simulink model "DatAnalysis"  (R2020a)
settings: Solver=FixedStepAuto  StartTime=0.0  StopTime=t_end  FixedStep=0.001  RelTol=1e-3
undefined symbols (not defined in the file or in its folder): DiscIntNeverNeededParam, Je, Ka, Ks, Le, We
libraries: simulink x6, dspstat3 x2, simulink_extras x2, dspsigops x2
settings Model: Creator=leona  LastModifiedBy=leona
settings DataIOCC: SaveFormat=StructureWithTime  SaveOutput=off  SignalLogging=off  DSMLogging=off  SaveTime=off  ReturnWorkspaceOutputs=off

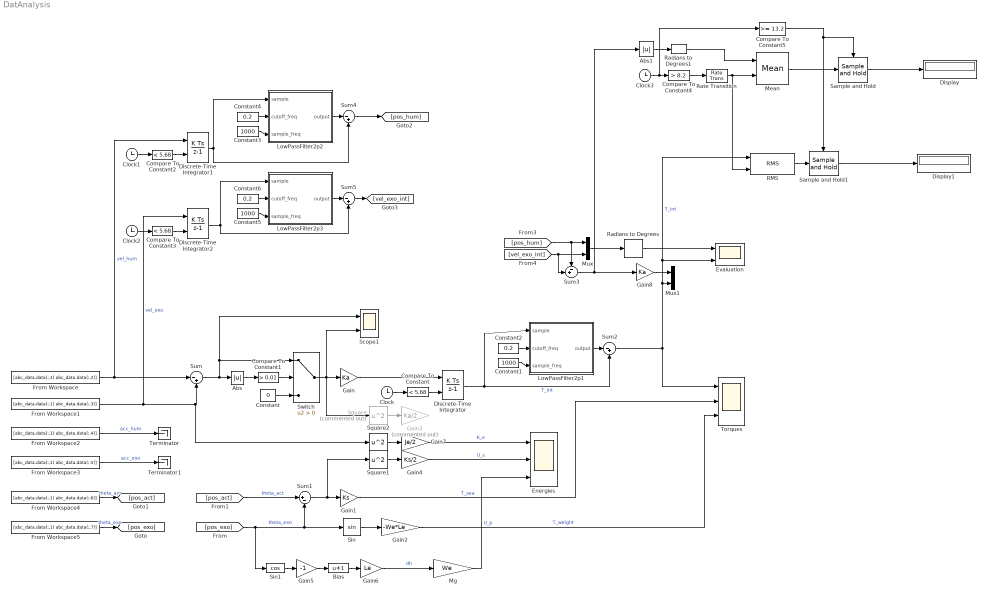
== system DatAnalysis ==
  Abs : Abs
  Abs1 : Abs
  Bias : Bias  Bias=1
  Clock{,1..3} (4 alike) : Clock
  Compare To Constant : simulink/Logic and Bit Operations/Compare To Constant  relop=<  const=5.68  OutDataTypeStr=boolean
  Compare To Constant1 : simulink/Logic and Bit Operations/Compare To Constant  relop=>  const=0.01  OutDataTypeStr=boolean
  Compare To Constant2 : simulink/Logic and Bit Operations/Compare To Constant  relop=<  const=5.68  OutDataTypeStr=boolean
  Compare To Constant3 : simulink/Logic and Bit Operations/Compare To Constant  relop=<  const=5.68  OutDataTypeStr=boolean
  Compare To Constant4 : simulink/Logic and Bit Operations/Compare To Constant  relop=>  const=8.2  OutDataTypeStr=boolean
  Compare To Constant5 : simulink/Logic and Bit Operations/Compare To Constant  relop=>=  const=13.2  OutDataTypeStr=boolean
  Constant : Constant  Value=0
  Constant1 : Constant  Value=1000
  Constant2 : Constant  Value=0.2
  Constant3 : Constant  Value=1000
  Constant4 : Constant  Value=0.2
  Constant5 : Constant  Value=1000
  Constant6 : Constant  Value=0.2
  Discrete-Time Integrator : DiscreteIntegrator  ExternalReset=level  SampleTime=0.001  ICPrevOutput=DiscIntNeverNeededParam  ICPrevScaledInput=DiscIntNeverNeededParam
  Discrete-Time Integrator1 : DiscreteIntegrator  ExternalReset=level  SampleTime=0.001  ICPrevOutput=DiscIntNeverNeededParam  ICPrevScaledInput=DiscIntNeverNeededParam
  Discrete-Time Integrator2 : DiscreteIntegrator  ExternalReset=level  SampleTime=0.001  ICPrevOutput=DiscIntNeverNeededParam  ICPrevScaledInput=DiscIntNeverNeededParam
  Display : Display
  Display1 : Display
  Energies : Scope  NumInputPorts=3
  Evaluation : Scope  NumInputPorts=2
  From Workspace : FromWorkspace  VariableName=[abc_data.data(:,1) abc_data.data(:,2)]  SampleTime=0.001  Interpolate=off  OutputAfterFinalValue=Holding final value
  From Workspace1 : FromWorkspace  VariableName=[abc_data.data(:,1) abc_data.data(:,3)]  SampleTime=0.001  Interpolate=off  OutputAfterFinalValue=Holding final value
  From Workspace2 : FromWorkspace  VariableName=[abc_data.data(:,1) abc_data.data(:,4)]  SampleTime=0.001  Interpolate=off  OutputAfterFinalValue=Holding final value
  From Workspace3 : FromWorkspace  VariableName=[abc_data.data(:,1) abc_data.data(:,5)]  SampleTime=0.001  Interpolate=off  OutputAfterFinalValue=Holding final value
  From Workspace4 : FromWorkspace  VariableName=[abc_data.data(:,1) abc_data.data(:,6)]  SampleTime=0.001  Interpolate=off  OutputAfterFinalValue=Holding final value
  From Workspace5 : FromWorkspace  VariableName=[abc_data.data(:,1) abc_data.data(:,7)]  SampleTime=0.001  Interpolate=off  OutputAfterFinalValue=Holding final value
  Gain : Gain  Gain=Ka
  Gain1 : Gain  Gain=Ks
  Gain2 : Gain  Gain=-We*Le
  Gain3 : Gain  Commented=on  Gain=Ka/2
  Gain4 : Gain  Gain=Ks/2
  Gain5 : Gain  Gain=-1
  Gain6 : Gain  Gain=Le
  Gain7 : Gain  Gain=Je/2
  Gain8 : Gain  Gain=Ka
  LowPassFilter2p1 : Subsystem
  LowPassFilter2p2 : Subsystem
  LowPassFilter2p3 : Subsystem
  Mean : dspstat3/Mean  run=on  InputProcessing=Columns as channels (frame based)  reset_popup=Rising edge  directionMode=Each column  dimension=1  roiEnable=off  roiType=Rectangles  roiPortion=Entire ROI  roiOutput=Individual statistics for each ROI  roiFlag=off  roundingMode=Floor  overflowMode=off  outputDataTypeStr=Inherit: Same as accumulator  outputMin=[]  outputMax=[]  outputLastDataTypeStr=Inherit: Same as accumulator
  Mg : Gain  Gain=We
  Mux : Mux  Inputs=2
  Mux1 : Mux  Inputs=2
  RMS : dspstat3/RMS  run=on  directionMode=Each column  dimension=1  InputProcessing=Columns as channels (frame based)  reset_popup=Rising edge
  Radians to Degrees : simulink_extras/Transformations/Radians to Degrees
  Radians to Degrees1 : simulink_extras/Transformations/Radians to Degrees
  Rate Transition : RateTransition  OutPortSampleTime=0.001
  Sample and Hold : dspsigops/Sample and Hold  trig=Rising edge  initCond=0  latchinput=off
  Sample and Hold1 : dspsigops/Sample and Hold  trig=Rising edge  initCond=0  latchinput=off
  Scope1 : Scope  NumInputPorts=2
  Sin : Trigonometry
  Sin1 : Trigonometry  Operator=cos
  Square : Math  Commented=on  Operator=square  SaturateOnIntegerOverflow=on
  Square1 : Math  Operator=square  SaturateOnIntegerOverflow=on
  Square2 : Math  Operator=square  SaturateOnIntegerOverflow=on
  Sum{,2,4..5} (4 alike) : Sum  Inputs=|-+
  Sum1 : Sum  Inputs=|+-
  Sum3 : Sum  Inputs=-+|
  Switch : Switch  Criteria=u2 > Threshold
  Terminator : Terminator
  Terminator1 : Terminator
  Torques : Scope  NumInputPorts=3
  wires:
  From Workspace/1 -> Sum/1, Discrete-Time Integrator1/1  "vel_hum"
  From Workspace1/1 -> Square2/1, Sum/2, Discrete-Time Integrator2/1  "vel_exo"
  Gain/1 -> Discrete-Time Integrator/1
  [pos_act] -> Sum1/1  "theta_act"
  [pos_exo] -> Sin1/1, Sum1/2, Sin/1  "theta_exo"
  Sum1/1 -> Square1/1, Gain1/1
  Sin/1 -> Gain2/1
  Gain2/1 -> Torques/3  "T_weight"
  From Workspace2/1 -> Terminator/1  "acc_hum"
  From Workspace3/1 -> Terminator1/1  "acc_exo"
  Clock/1 -> Compare To Constant/1
  Compare To Constant/1 -> Discrete-Time Integrator/2
  Switch/1 -> Scope1/2, Square/1, Gain/1
  Sum/1 -> Abs/1, Switch/1, Scope1/1
  Compare To Constant1/1 -> Switch/2
  Abs/1 -> Compare To Constant1/1
  Constant/1 -> Switch/3
  LowPassFilter2p1/1(output) -> Sum2/1
  Discrete-Time Integrator/1 -> LowPassFilter2p1/1(sample), Sum2/2  "T_int"
  Constant1/1 -> LowPassFilter2p1/3(sample_freq)
  Constant2/1 -> LowPassFilter2p1/2(cutoff_freq)
  Sum2/1 -> Evaluation/2, RMS/1, Mux1/2, Torques/1  "T_int"
  Gain1/1 -> Torques/2  "T_sea"
  Square/1 -> Gain3/1
  Square1/1 -> Gain4/1
  Gain4/1 -> Energies/2  "U_s"
  Gain6/1 -> Mg/1  "dh"
  Mg/1 -> Energies/3  "U_p"
  Sin1/1 -> Gain5/1
  Gain5/1 -> Bias/1
  Bias/1 -> Gain6/1
  Square2/1 -> Gain7/1
  Gain7/1 -> Energies/1  "K_e"
  Compare To Constant2/1 -> Discrete-Time Integrator1/2
  Clock1/1 -> Compare To Constant2/1
  Mux/1 -> Radians to Degrees/1
  From Workspace5/1 -> [pos_exo]  "theta_exo"
  From Workspace4/1 -> [pos_act]  "theta_act"
  Radians to Degrees/1 -> Evaluation/1
  [pos_hum] -> Sum3/1, Mux/1
  Gain8/1 -> Mux1/1
  Clock2/1 -> Compare To Constant3/1
  Compare To Constant3/1 -> Discrete-Time Integrator2/2
  [vel_exo_int] -> Sum3/2, Mux/2
  Constant4/1 -> LowPassFilter2p2/2(cutoff_freq)
  Constant3/1 -> LowPassFilter2p2/3(sample_freq)
  Discrete-Time Integrator1/1 -> LowPassFilter2p2/1(sample), Sum4/2
  LowPassFilter2p2/1(output) -> Sum4/1
  Sum4/1 -> [pos_hum]
  Discrete-Time Integrator2/1 -> LowPassFilter2p3/1(sample), Sum5/2
  Constant5/1 -> LowPassFilter2p3/3(sample_freq)
  Constant6/1 -> LowPassFilter2p3/2(cutoff_freq)
  LowPassFilter2p3/1(output) -> Sum5/1
  Sum5/1 -> [vel_exo_int]
  Clock3/1 -> Compare To Constant5/1, Compare To Constant4/1
  Compare To Constant4/1 -> Rate Transition/1
  Abs1/1 -> Radians to Degrees1/1
  Radians to Degrees1/1 -> Mean/1
  Mean/1 -> Sample and Hold/1
  Compare To Constant5/1 -> Sample and Hold/Trigger, Sample and Hold1/Trigger
  Sample and Hold/1 -> Display/1
  Sum3/1 -> Abs1/1, Gain8/1
  Rate Transition/1 -> Mean/2, RMS/2
  Sample and Hold1/1 -> Display1/1
  RMS/1 -> Sample and Hold1/1

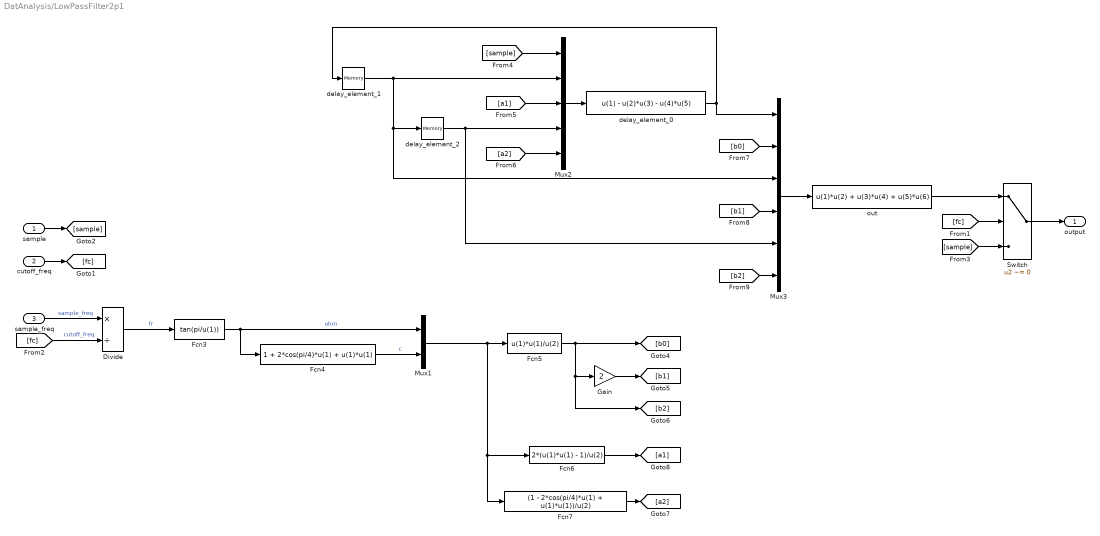
== system DatAnalysis/LowPassFilter2p1 ==
  sample : Inport
  cutoff_freq : Inport  Port=2
  sample_freq : Inport  Port=3
  Divide : Product  Inputs=*/
  Fcn3 : Fcn  Expr=tan(pi/u(1))
  Fcn4 : Fcn  Expr=1 + 2*cos(pi/4)*u(1) + u(1)*u(1)
  Fcn5 : Fcn  Expr=u(1)*u(1)/u(2)
  Fcn6 : Fcn  Expr=2*(u(1)*u(1) - 1)/u(2)
  Fcn7 : Fcn  Expr=(1 - 2*cos(pi/4)*u(1) + u(1)*u(1))/u(2)
  Gain : Gain  Gain=2
  Mux1 : Mux  Inputs=2
  Mux2 : Mux  Inputs=5
  Mux3 : Mux  Inputs=6
  Switch : Switch  Criteria=u2 ~= 0
  delay_element_0 : Fcn  Expr=u(1) - u(2)*u(3) - u(4)*u(5)
  delay_element_1 : Memory  InheritSampleTime=on
  delay_element_2 : Memory  InheritSampleTime=on
  out : Fcn  Expr=u(1)*u(2) + u(3)*u(4) + u(5)*u(6)
  output : Outport
  wires:
  Mux3/1 -> out/1
  [b2] -> Mux3/6
  [b1] -> Mux3/4
  [b0] -> Mux3/2
  delay_element_0/1 -> Mux3/1, delay_element_1/1
  out/1 -> Switch/1
  [a2] -> Mux2/5
  delay_element_2/1 -> Mux3/5, Mux2/4
  [a1] -> Mux2/3
  Mux2/1 -> delay_element_0/1
  [sample] -> Mux2/1
  delay_element_1/1 -> Mux2/2, Mux3/3, delay_element_2/1
  [sample] -> Switch/3
  sample/1 -> [sample]
  Fcn7/1 -> [a2]
  Fcn6/1 -> [a1]
  Gain/1 -> [b1]
  Fcn5/1 -> Gain/1, [b2], [b0]
  Fcn4/1 -> Mux1/2  "c"
  Fcn3/1 -> Fcn4/1, Mux1/1  "ohm"
  Mux1/1 -> Fcn5/1, Fcn6/1, Fcn7/1
  Divide/1 -> Fcn3/1  "fr"
  [fc] -> Divide/2  "cutoff_freq"
  sample_freq/1 -> Divide/1  "sample_freq"
  [fc] -> Switch/2
  cutoff_freq/1 -> [fc]
  Switch/1 -> output/1

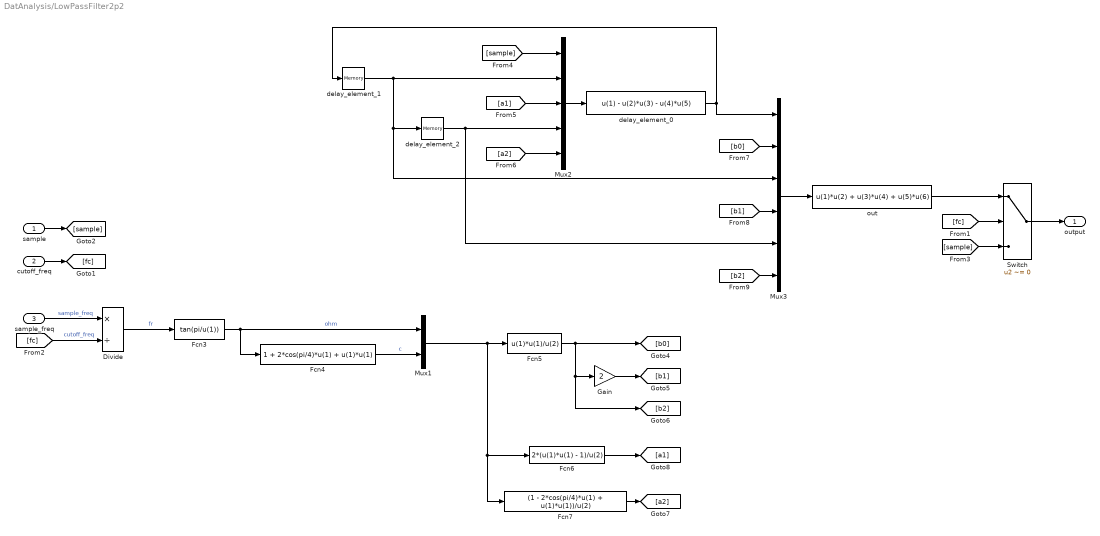
== system DatAnalysis/LowPassFilter2p2 ==
  sample : Inport
  cutoff_freq : Inport  Port=2
  sample_freq : Inport  Port=3
  Divide : Product  Inputs=*/
  Fcn3 : Fcn  Expr=tan(pi/u(1))
  Fcn4 : Fcn  Expr=1 + 2*cos(pi/4)*u(1) + u(1)*u(1)
  Fcn5 : Fcn  Expr=u(1)*u(1)/u(2)
  Fcn6 : Fcn  Expr=2*(u(1)*u(1) - 1)/u(2)
  Fcn7 : Fcn  Expr=(1 - 2*cos(pi/4)*u(1) + u(1)*u(1))/u(2)
  Gain : Gain  Gain=2
  Mux1 : Mux  Inputs=2
  Mux2 : Mux  Inputs=5
  Mux3 : Mux  Inputs=6
  Switch : Switch  Criteria=u2 ~= 0
  delay_element_0 : Fcn  Expr=u(1) - u(2)*u(3) - u(4)*u(5)
  delay_element_1 : Memory  InheritSampleTime=on
  delay_element_2 : Memory  InheritSampleTime=on
  out : Fcn  Expr=u(1)*u(2) + u(3)*u(4) + u(5)*u(6)
  output : Outport
  wires:
  Switch/1 -> output/1
  cutoff_freq/1 -> [fc]
  [fc] -> Switch/2
  sample_freq/1 -> Divide/1  "sample_freq"
  [fc] -> Divide/2  "cutoff_freq"
  Divide/1 -> Fcn3/1  "fr"
  Mux1/1 -> Fcn7/1, Fcn6/1, Fcn5/1
  Fcn3/1 -> Mux1/1, Fcn4/1  "ohm"
  Fcn4/1 -> Mux1/2  "c"
  Fcn5/1 -> [b0], [b2], Gain/1
  Gain/1 -> [b1]
  Fcn6/1 -> [a1]
  Fcn7/1 -> [a2]
  sample/1 -> [sample]
  [sample] -> Switch/3
  delay_element_1/1 -> delay_element_2/1, Mux3/3, Mux2/2
  [sample] -> Mux2/1
  Mux2/1 -> delay_element_0/1
  [a1] -> Mux2/3
  delay_element_2/1 -> Mux2/4, Mux3/5
  [a2] -> Mux2/5
  out/1 -> Switch/1
  delay_element_0/1 -> delay_element_1/1, Mux3/1
  [b0] -> Mux3/2
  [b1] -> Mux3/4
  [b2] -> Mux3/6
  Mux3/1 -> out/1

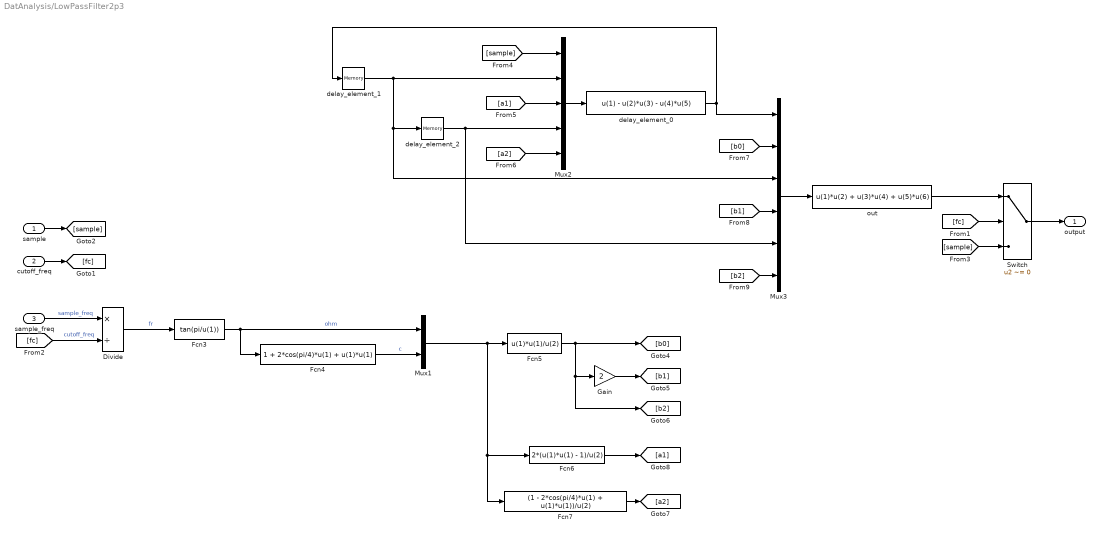
== system DatAnalysis/LowPassFilter2p3 ==
  sample : Inport
  cutoff_freq : Inport  Port=2
  sample_freq : Inport  Port=3
  Divide : Product  Inputs=*/
  Fcn3 : Fcn  Expr=tan(pi/u(1))
  Fcn4 : Fcn  Expr=1 + 2*cos(pi/4)*u(1) + u(1)*u(1)
  Fcn5 : Fcn  Expr=u(1)*u(1)/u(2)
  Fcn6 : Fcn  Expr=2*(u(1)*u(1) - 1)/u(2)
  Fcn7 : Fcn  Expr=(1 - 2*cos(pi/4)*u(1) + u(1)*u(1))/u(2)
  Gain : Gain  Gain=2
  Mux1 : Mux  Inputs=2
  Mux2 : Mux  Inputs=5
  Mux3 : Mux  Inputs=6
  Switch : Switch  Criteria=u2 ~= 0
  delay_element_0 : Fcn  Expr=u(1) - u(2)*u(3) - u(4)*u(5)
  delay_element_1 : Memory  InheritSampleTime=on
  delay_element_2 : Memory  InheritSampleTime=on
  out : Fcn  Expr=u(1)*u(2) + u(3)*u(4) + u(5)*u(6)
  output : Outport
  wires:
  Mux3/1 -> out/1
  [b2] -> Mux3/6
  [b1] -> Mux3/4
  [b0] -> Mux3/2
  delay_element_0/1 -> Mux3/1, delay_element_1/1
  out/1 -> Switch/1
  [a2] -> Mux2/5
  delay_element_2/1 -> Mux3/5, Mux2/4
  [a1] -> Mux2/3
  Mux2/1 -> delay_element_0/1
  [sample] -> Mux2/1
  delay_element_1/1 -> Mux2/2, Mux3/3, delay_element_2/1
  [sample] -> Switch/3
  sample/1 -> [sample]
  Fcn7/1 -> [a2]
  Fcn6/1 -> [a1]
  Gain/1 -> [b1]
  Fcn5/1 -> Gain/1, [b2], [b0]
  Fcn4/1 -> Mux1/2  "c"
  Fcn3/1 -> Fcn4/1, Mux1/1  "ohm"
  Mux1/1 -> Fcn5/1, Fcn6/1, Fcn7/1
  Divide/1 -> Fcn3/1  "fr"
  [fc] -> Divide/2  "cutoff_freq"
  sample_freq/1 -> Divide/1  "sample_freq"
  [fc] -> Switch/2
  cutoff_freq/1 -> [fc]
  Switch/1 -> output/1
